simulink model "bp2_model"  (R2022a)
settings: Solver=ode15s  StartTime=0.0  StopTime=5000  RelTol=3e-14  EnableMultiTasking=on
PreLoadFcn:
  | ww=[1e-7 1e6]; N=41;
libraries: cstblocks x2
settings Model: Creator=Dingyu  LastModifiedBy=xuedi
settings SolverCC: AlgebraicLoopSolver=TrustRegion
settings DataIOCC: SaveFormat=Array  ReturnWorkspaceOutputs=off
settings OptimizationCC: LifeSpan=inf
settings DebuggingCC: UnconnectedInputMsg=warning  UnconnectedOutputMsg=warning  UnconnectedLineMsg=warning  SFUnexpectedBacktrackingDiag=warning  SFNoUnconditionalDefaultTransitionDiag=warning  SFExecutionAtInitializationDiag=none  SFMachineParentedDataDiag=warning  ArithmeticOperatorsInVariantConditions=warning
settings SFSimCC: SimUseLocalCustomCode=off  CustomCodeUndefinedFunction=UseInterfaceOnly
settings RTWCC: RTWUseLocalCustomCode=off  DLArmComputeVersion=19.05
settings CodeAppCC: StateflowObjectComments=on
settings GRTTargetCC: TargetLangStandard=C89/C90 (ANSI)
settings ConfigComp: CovMetricSettings=dw  CovSaveCumulativeToWorkspaceVar=on  CovSaveSingleToWorkspaceVar=on  CovExternalEMLEnable=off

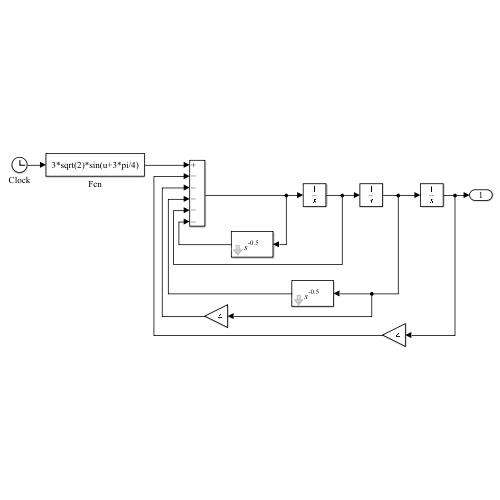
[thumbnail: Simulink's stored preview of the top-level diagram]
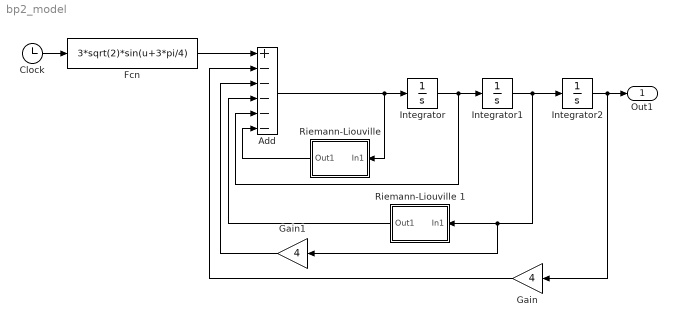
== system bp2_model ==
  Add : Sum  Inputs=+-----
  Clock : Clock
  Fcn : Fcn  Expr=3*sqrt(2)*sin(u+3*pi/4)
  Gain : Gain  Gain=4
  Gain1 : Gain  Gain=4
  Integrator : Integrator  InitialCondition=-1
  Integrator1 : Integrator
  Integrator2 : Integrator  InitialCondition=1
  "Riemann-Liouville " : Subsystem  mask{gam=-0.5, ww=ww, n=N, kF1=on, kF=Oustaloup filter}
      mask prompts: gam "Derivative order gamma"; ww "Frequency range [wb,wh]"; n "Apprixmation order"; kF1 "Is a low-pass filter required?"; kF "Filter type"
      mask init:
      | wb=ww(1); wh=ww(2); 
      |    if isnumeric(gam), str=['{\its}^{' num2str(gam) '}']; 
      |    else, str='{\its}^{\gamma}'; end
      |    switch kF
      |       case 1, G=ousta_fod(gam,n,wb,wh);
      |       case 2, G=new_fod(gam,n,wb,wh); 
      |       case 3, G=matsuda_fod(gam,n,wb,wh); 
      |       case 4, G=srid_fod(gam,0.01,n);
      |    end
      |    T=1e-6/wh; if kF1==1, G=G*tf(1,[T 1]); end
      mask TypeOptions kF: Oustaloup filter | Modified Oustaloup filter | Matsuda-Fujii filter | Discrete step invariant filter
      mask Display: disp(str,'texmode','on')
  Riemann-Liouville 1 : Subsystem  mask{gam=-0.5, ww=ww, n=N, kF1=off, kF=Oustaloup filter}
      mask prompts: gam "Derivative order gamma"; ww "Frequency range [wb,wh]"; n "Apprixmation order"; kF1 "Is a low-pass filter required?"; kF "Filter type"
      mask init: same as bp2_model/Riemann-Liouville 
      mask TypeOptions kF: Oustaloup filter | Modified Oustaloup filter | Matsuda-Fujii filter | Discrete step invariant filter
      mask Display: disp(str,'texmode','on')
  Out1 : Outport
  wires:
  Integrator2/1 -> Out1/1, Gain/1
  Gain/1 -> Add/2
  Clock/1 -> Fcn/1
  Fcn/1 -> Add/1
  Integrator/1 -> Add/5, Integrator1/1
  Gain1/1 -> Add/3
  Add/1 -> "Riemann-Liouville "/1(In1), Integrator/1
  Integrator1/1 -> Integrator2/1, Riemann-Liouville 1/1(In1), Gain1/1
  "Riemann-Liouville "/1(Out1) -> Add/6
  Riemann-Liouville 1/1(Out1) -> Add/4

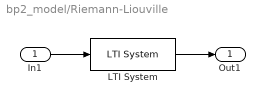
== system bp2_model/Riemann-Liouville  ==
  In1 : Inport
  LTI System : cstblocks/LTI System  sys=G  IC=[]
  Out1 : Outport
  wires:
  LTI System/1 -> Out1/1
  In1/1 -> LTI System/1

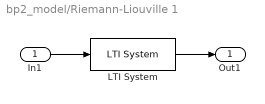
== system bp2_model/Riemann-Liouville 1 ==
  In1 : Inport
  LTI System : cstblocks/LTI System  sys=G  IC=[]
  Out1 : Outport
  wires:
  In1/1 -> LTI System/1
  LTI System/1 -> Out1/1
